simulink model "StateFlows_RevF"  (R2020a)
settings: Solver=FixedStepAuto  StartTime=0.0  StopTime=10.0  FixedStep=1e-3  RelTol=1e-3  EnableMultiTasking=on
undefined symbols (not defined in the file): A0, A1, D0, D1, D10, D11, D12, D13, D2, D3, D5, D6, D8, D9, PTA0, PTA1, PTA2, PTB2, PTB3, PTB9, PTC16, PTC17, PTC2, PTC4, PTD0, PTD1, PTD2, PTD3
libraries: frdmk64flib x17, etargetslib x13, dspstat3 x1
settings Model: ExtModeTrigDuration=5  Creator=dexho  LastModifiedBy=dexho
settings OptimizationCC: EnhancedBackFolding=on  PassReuseOutputArgsAs=Individual arguments  ZeroExternalMemoryAtStartup=off  ZeroInternalMemoryAtStartup=off  MaxStackSize=64  OptimizeBlockOrder=speed  DifferentSizesBufferReuse=on  OptimizationCustomize=off  EfficientTunableParamExpr=on
settings DebuggingCC: ParameterTunabilityLossMsg=error  UnconnectedInputMsg=none  UnconnectedOutputMsg=none  UnconnectedLineMsg=none
settings HardwareCC: ProdBitPerPointer=32  ProdBitPerSizeT=32  ProdBitPerPtrDiffT=32  ProdLargestAtomicInteger=Long  ProdLargestAtomicFloat=Double  ProdWordSize=32  ProdHWDeviceType=ARM Compatible->ARM Cortex
settings ModelReferenceCC: EnableRefExpFcnMdlSchedulingChecks=off
settings SFSimCC: MATLABDynamicMemAlloc=off
settings RTWCC: SystemTargetFile=ert.tlc  HardwareBoard=NXP FRDM-K64F  TemplateMakefile=ert_default_tmf  Toolchain=GNU Tools for ARM Embedded Processors
settings CodeAppCC: ForceParamTrailComments=on  IgnoreCustomStorageClasses=off  OperatorAnnotations=on  SimulinkDataObjDesc=on  SFDataObjDesc=on  InsertBlockDesc=on
settings ERTTargetCC: ExtModeTransport=4  ExtModeMexFile=sendToCommService

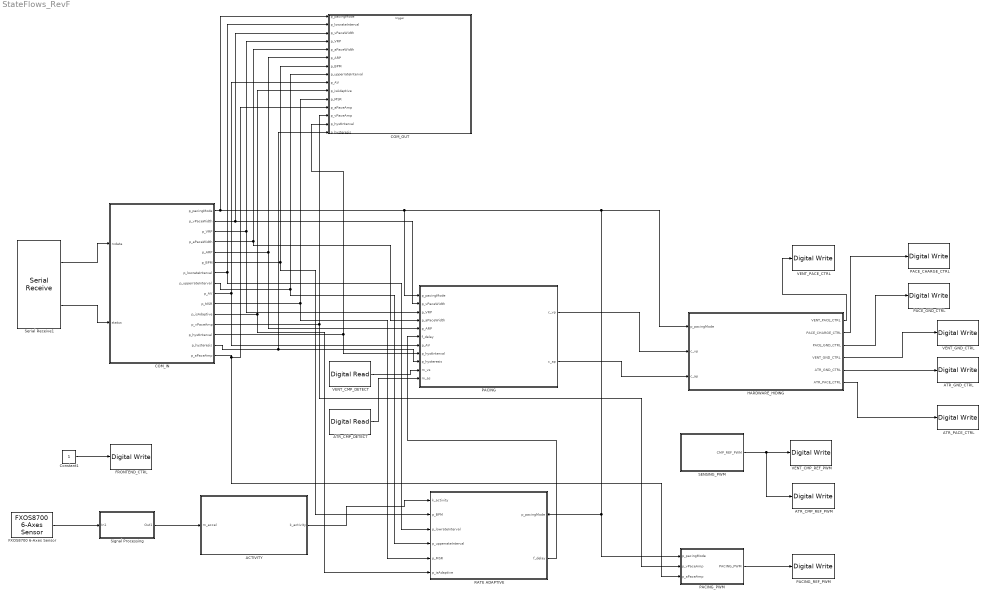
== system StateFlows_RevF ==
  ACTIVITY : Stateflow chart  TreatAsAtomicUnit=on
  ATR_CMP_DETECT : frdmk64flib/Digital Read  Whichpin=PTC16 (D0)  SampleTime=-1
  ATR_CMP_REF_PWM : frdmk64flib/Digital Write  Whichpin=PTC2 (D6)
  ATR_GND_CTRL : frdmk64flib/Digital Write  Whichpin=PTD2 (D11)
  ATR_PACE_CTRL : frdmk64flib/Digital Write  Whichpin=PTA0 (D8)
  COM_IN : Stateflow chart  TreatAsAtomicUnit=on
      settings: PortSchema="{\"entries\":[{\"content\":{\"sides\":[{\"content\":{\"connectorIds\":[\"In1\",\"In2\"]},\"type\":\"ConnectorPlacement.EquallySpacedRectSide\",\"uuid\":\"4343c62c-52df-4cc9-ac4a-2b1e5390f7dd\"},{\"content\":{\"connectorIds\":[\"Out1\",\"Out3\",\"Out4\",\"Out5\",\"Out6\",\"Out7\",\"Out2\",\"Out8\",\"Out9\",\"Out11\",\"Out10\",\"Out13\",\"Out14\",\"Out15\",\"Out12\"],\"side\":\"RIGHT\"},\"type\":\"ConnectorPlacement.EquallySpacedRectSide\",\"uuid\":\"27c89a21-e9bb-4d00-a5b8-19e687f961a4\"},{\"content\":{\"connectorIds\":[],\"side\":\"TOP\"},\"type\":\"ConnectorPlacement.EquallySpacedRectSide\",\"uuid\":\"0da42faa-8fe8-4994-9d32-ed3ce1a64f57\"}]},\"type\":\"ConnectorPlacement.EquallySpacedConnector\",\"uuid\":\"30cce4c4-f2f2-4d0d-92ef-56531670e1a1\"}],\"packageUris\":[\"http://schema.mathworks.com/mf0/Connector/19700101\"],\"version\":\"1.0\"}"
  COM_OUT : Subsystem
  Constant1 : Constant
  FRONTEND_CTRL : frdmk64flib/Digital Write  Whichpin=PTD1 (D13)
  FXOS8700 6-Axes Sensor : frdmk64flib/FXOS8700 6-Axes Sensor  Activesensor=Accelerometer only  ODR=100Hz  HybridODR=400Hz  Accelfullrange=-4g to +4g  SampleTime=-1
  HARDWARE_HIDING : Stateflow chart  TreatAsAtomicUnit=on
  PACE_CHARGE_CTRL : frdmk64flib/Digital Write  Whichpin=PTB9 (D2)
  PACE_GND_CTRL : frdmk64flib/Digital Write  Whichpin=PTD0 (D10)
  PACING : Stateflow chart  TreatAsAtomicUnit=on
      settings: PortSchema="{\"entries\":[{\"content\":{\"sides\":[{\"content\":{\"connectorIds\":[\"In3\",\"In4\",\"In5\",\"In6\",\"In7\",\"In8\",\"In9\",\"In10\",\"In11\",\"In1\",\"In2\"]},\"type\":\"ConnectorPlacement.EquallySpacedRectSide\",\"uuid\":\"abf03a48-0fa7-45c4-991f-e42ac80c6e9f\"},{\"content\":{\"connectorIds\":[\"Out1\",\"Out2\"],\"side\":\"RIGHT\"},\"type\":\"ConnectorPlacement.EquallySpacedRectSide\",\"uuid\":\"03e9df7b-3413-4ae5-9bc1-782036bbbe85\"},{\"content\":{\"connectorIds\":[],\"side\":\"TOP\"},\"type\":\"ConnectorPlacement.EquallySpacedRectSide\",\"uuid\":\"2119f2bc-1283-45d3-ae9d-33c8aada0ca6\"}]},\"type\":\"ConnectorPlacement.EquallySpacedConnector\",\"uuid\":\"89ff8e32-b874-4b74-b5d9-0aa878838f6d\"}],\"packageUris\":[\"http://schema.mathworks.com/mf0/Connector/19700101\"],\"version\":\"1.0\"}"
  PACING_PWM : Stateflow chart  TreatAsAtomicUnit=on
  PACING_REF_PWM : frdmk64flib/Digital Write  Whichpin=PTA2 (D5)
  RATE ADAPTIVE : Stateflow chart  TreatAsAtomicUnit=on
      settings: PortSchema="{\"entries\":[{\"content\":{\"sides\":[{\"content\":{\"connectorIds\":[\"In1\",\"In2\",\"In3\",\"In5\",\"In6\",\"In7\"]},\"type\":\"ConnectorPlacement.EquallySpacedRectSide\",\"uuid\":\"970c8990-33da-4b83-8419-4bdc08160303\"},{\"content\":{\"connectorIds\":[\"In4\",\"Out1\"],\"side\":\"RIGHT\"},\"type\":\"ConnectorPlacement.EquallySpacedRectSide\",\"uuid\":\"a18c4a49-244c-415b-8dfc-e199cb33ce07\"},{\"content\":{\"side\":\"TOP\"},\"type\":\"ConnectorPlacement.EquallySpacedRectSide\",\"uuid\":\"633c22bc-82ca-4f35-91f5-3ea1e9c4e467\"}]},\"type\":\"ConnectorPlacement.EquallySpacedConnector\",\"uuid\":\"9415645b-fdd6-4720-89a1-dcdad790b939\"}],\"packageUris\":[\"http://schema.mathworks.com/mf0/Connector/R2020b\"],\"version\":\"1.0\"}"
  SENSING_PWM : Stateflow chart  TreatAsAtomicUnit=on
  Serial Receive1 : frdmk64flib/Serial Receive  SCIModule=0  Baudrate=uint32(9600)  Parity=None  StopBits=1  HardwareFlowControl=None  ByteOrder=LittleEndian  DataType=uint8  DataLength=46  BlockingMode=off  OutputStatus=on  SampleTime=-1
  Signal Processing : Subsystem
  VENT_CMP_DETECT : frdmk64flib/Digital Read  Whichpin=PTC17 (D1)  SampleTime=-1
  VENT_CMP_REF_PWM : frdmk64flib/Digital Write  Whichpin=PTA1 (D3)
  VENT_GND_CTRL : frdmk64flib/Digital Write  Whichpin=PTD3 (D12)
  VENT_PACE_CTRL : frdmk64flib/Digital Write  Whichpin=PTC4 (D9)
  wires:
  VENT_CMP_DETECT/1 -> PACING/1(m_vs)
  ATR_CMP_DETECT/1 -> PACING/2(m_as)
  Constant1/1 -> FRONTEND_CTRL/1
  PACING_PWM/1(PACING_PWM) -> PACING_REF_PWM/1
  SENSING_PWM/1(CMP_REF_PWM) -> ATR_CMP_REF_PWM/1, VENT_CMP_REF_PWM/1
  COM_IN/1(p_pacingMode) -> COM_OUT/1(p_pacingMode), PACING/3(p_pacingMode), HARDWARE_HIDING/1(p_pacingMode), PACING_PWM/1(p_pacingMode), RATE ADAPTIVE/4(p_pacingMode)
  PACING/1(c_vp) -> HARDWARE_HIDING/2(c_vp)
  PACING/2(c_ap) -> HARDWARE_HIDING/3(c_ap)
  HARDWARE_HIDING/1(VENT_PACE_CTRL) -> VENT_PACE_CTRL/1
  HARDWARE_HIDING/2(PACE_CHARGE_CTRL) -> PACE_CHARGE_CTRL/1
  HARDWARE_HIDING/3(PACE_GND_CTRL) -> PACE_GND_CTRL/1
  HARDWARE_HIDING/4(VENT_GND_CTRL) -> VENT_GND_CTRL/1
  HARDWARE_HIDING/5(ATR_GND_CTRL) -> ATR_GND_CTRL/1
  HARDWARE_HIDING/6(ATR_PACE_CTRL) -> ATR_PACE_CTRL/1
  Signal Processing/1(Out1) -> ACTIVITY/1(m_accel)
  FXOS8700 6-Axes Sensor/1 -> Signal Processing/1(In1)
  ACTIVITY/1(k_activity) -> RATE ADAPTIVE/1(k_activity)
  RATE ADAPTIVE/1(f_delay) -> PACING/8(f_delay)
  Serial Receive1/1 -> COM_IN/1(rxdata)
  Serial Receive1/2 -> COM_IN/2(status)
  COM_IN/3(p_vPaceWidth) -> COM_OUT/3(p_vPaceWidth), PACING/4(p_vPaceWidth)
  COM_IN/4(p_VRP) -> PACING/5(p_VRP), COM_OUT/4(p_VRP)
  COM_IN/5(p_aPaceWidth) -> PACING/6(p_aPaceWidth), COM_OUT/5(p_aPaceWidth)
  COM_IN/6(p_ARP) -> PACING/7(p_ARP), COM_OUT/6(p_ARP)
  COM_IN/9(p_AV) -> PACING/9(p_AV), COM_OUT/9(p_AV)
  COM_IN/11(p_MSR) -> RATE ADAPTIVE/6(p_MSR), COM_OUT/11(p_MSR)
  COM_IN/10(p_isAdaptive) -> RATE ADAPTIVE/7(p_isAdaptive), COM_OUT/10(p_isAdaptive)
  COM_IN/8(p_upperrateInterval) -> RATE ADAPTIVE/5(p_upperrateInterval), COM_OUT/8(p_upperrateInterval)
  COM_IN/2(p_lowrateInterval) -> RATE ADAPTIVE/3(p_lowrateInterval), COM_OUT/2(p_lowrateInterval)
  COM_IN/7(p_BPM) -> RATE ADAPTIVE/2(p_BPM), COM_OUT/7(p_BPM)
  COM_IN/13(p_vPaceAmp) -> PACING_PWM/2(p_vPaceAmp), COM_OUT/13(p_vPaceAmp)
  COM_IN/12(p_aPaceAmp) -> PACING_PWM/3(p_aPaceAmp), COM_OUT/12(p_aPaceAmp)
  COM_IN/14(p_hystInterval) -> PACING/10(p_hystInterval), COM_OUT/14(p_hystInterval)
  COM_IN/15(p_hysteresis) -> COM_OUT/15(p_hysteresis), PACING/11(p_hysteresis)

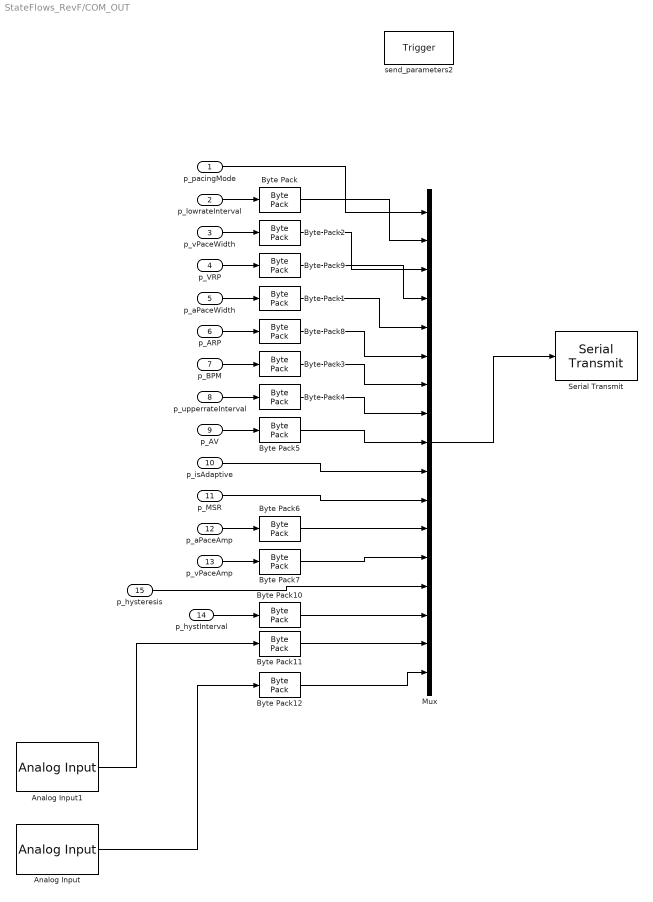
== system StateFlows_RevF/COM_OUT ==
  p_pacingMode : Inport  OutDataTypeStr=uint8
  p_lowrateInterval : Inport  Port=2  OutDataTypeStr=single
  p_vPaceWidth : Inport  Port=3  OutDataTypeStr=single
  p_VRP : Inport  Port=4  OutDataTypeStr=uint16
  p_aPaceWidth : Inport  Port=5  OutDataTypeStr=single
  p_ARP : Inport  Port=6  OutDataTypeStr=uint16
  p_BPM : Inport  Port=7  OutDataTypeStr=single
  p_upperrateInterval : Inport  Port=8  OutDataTypeStr=single
  p_AV : Inport  Port=9  OutDataTypeStr=single
  p_isAdaptive : Inport  Port=10  OutDataTypeStr=uint8
  p_MSR : Inport  Port=11  OutDataTypeStr=uint8
  p_aPaceAmp : Inport  Port=12  OutDataTypeStr=single
  p_vPaceAmp : Inport  Port=13  OutDataTypeStr=single
  p_hystInterval : Inport  Port=14  OutDataTypeStr=single
  p_hysteresis : Inport  Port=15  OutDataTypeStr=uint8
  send_parameters2 : TriggerPort  TriggerType=function-call  IsSimulinkFunction=on  FunctionName=send_parameters2  VariantControl=(inherit)  PortDimensions=1
  Analog Input : frdmk64flib/Analog Input  Whichpin=PTB2 (A0)  SampleTime=-1
  Analog Input1 : frdmk64flib/Analog Input  Whichpin=PTB3 (A1)  SampleTime=-1
  Byte Pack{,1..7,10} (9 alike) : etargetslib/Byte Pack  datatypes={'single'}  byteAlign=1
  Byte Pack11 : etargetslib/Byte Pack  datatypes={'double'}  byteAlign=1
  Byte Pack12 : etargetslib/Byte Pack  datatypes={'double'}  byteAlign=1
  Byte Pack8 : etargetslib/Byte Pack  datatypes={'uint16'}  byteAlign=1
  Byte Pack9 : etargetslib/Byte Pack  datatypes={'uint16'}  byteAlign=1
  Mux : Mux  Inputs=17
  Serial Transmit : frdmk64flib/Serial Transmit  SCIModule=0  Baudrate=uint32(9600)  Parity=None  StopBits=1  HardwareFlowControl=None  ByteOrder=LittleEndian  BlockingMode=on  OutputStatus=off
  wires:
  Mux/1 -> Serial Transmit/1
  p_pacingMode/1 -> Mux/1
  p_lowrateInterval/1 -> Byte Pack/1
  p_vPaceWidth/1 -> Byte Pack2/1
  p_VRP/1 -> Byte Pack9/1
  p_aPaceWidth/1 -> Byte Pack1/1
  p_ARP/1 -> Byte Pack8/1
  p_BPM/1 -> Byte Pack3/1
  p_upperrateInterval/1 -> Byte Pack4/1
  p_AV/1 -> Byte Pack5/1
  p_aPaceAmp/1 -> Byte Pack6/1
  p_vPaceAmp/1 -> Byte Pack7/1
  Byte Pack/1 -> Mux/2
  Byte Pack2/1 -> Mux/3
  Byte Pack9/1 -> Mux/4
  Byte Pack1/1 -> Mux/5
  Byte Pack8/1 -> Mux/6
  Byte Pack3/1 -> Mux/7
  Byte Pack4/1 -> Mux/8
  Byte Pack5/1 -> Mux/9
  p_isAdaptive/1 -> Mux/10
  p_MSR/1 -> Mux/11
  Byte Pack6/1 -> Mux/12
  Byte Pack7/1 -> Mux/13
  p_hystInterval/1 -> Byte Pack10/1
  Byte Pack10/1 -> Mux/15
  Byte Pack11/1 -> Mux/16
  Byte Pack12/1 -> Mux/17
  Analog Input/1 -> Byte Pack12/1
  Analog Input1/1 -> Byte Pack11/1
  p_hysteresis/1 -> Mux/14

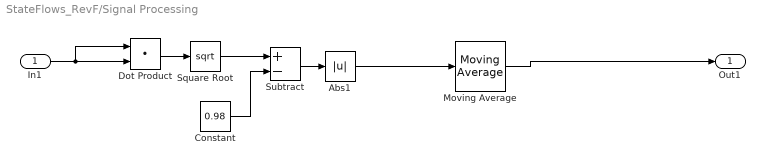
== system StateFlows_RevF/Signal Processing ==
  In1 : Inport
  Abs1 : Abs  OutDataTypeStr=double
  Constant : Constant  Value=0.98  OutDataTypeStr=double
  Dot Product : DotProduct  OutDataTypeStr=double  InputSameDT=on
  Moving Average : dspstat3/Moving Average  Method=Exponential weighting  ForgettingFactorPort=off  SpecifyWindowLength=on  WindowLength=4  ForgettingFactor=0.94  SimulateUsing=Code generation
  Square Root : Sqrt  OutputSignalType=real  OutDataTypeStr=double  SaturateOnIntegerOverflow=on
  Subtract : Sum  Inputs=+-
  Out1 : Outport  OutDataTypeStr=double
  wires:
  Constant/1 -> Subtract/2
  In1/1 -> Dot Product/2, Dot Product/1
  Subtract/1 -> Abs1/1
  Square Root/1 -> Subtract/1
  Dot Product/1 -> Square Root/1
  Abs1/1 -> Moving Average/1
  Moving Average/1 -> Out1/1

== stateflow chart StateFlows_RevF/SENSING_PWM ==
  state ON
    entry:
    CMP_REF_PWM = true;
  state OFF
    entry:
    CMP_REF_PWM = false;
  (default) -> ON
  ON -> OFF : [after((1000/freq)*0.8, msec)]
  OFF -> ON : [after((1000/freq)*0.2, msec)]
  data: CMP_REF_PWM output boolean; freq local double =200

== stateflow chart StateFlows_RevF/PACING_PWM ==
  state INIT
    entry:
    if(p_pacingMode == 0 || p_pacingMode == 2)
    f_dc = p_vPaceAmp / 5000;
    else
    f_dc = p_aPaceAmp / 5000;
    end
  state ON
    entry:
    PACING_PWM = true;
  state OFF
    entry:
    PACING_PWM = false;
  (default) -> INIT
  INIT -> ON
  ON -> OFF : [after((1000.0/freq)*f_dc, msec)]
  OFF -> ON : [after((1000.0/freq)*(1 - f_dc), msec)]
  data: PACING_PWM output boolean; freq local double =2000; p_pacingMode input uint8; p_vPaceAmp input single; p_aPaceAmp input single; f_dc local

== stateflow chart StateFlows_RevF/PACING ==
  state INIT
    entry:
    k_isHyst = 0;
  state CHARGE_DISCHARGE
    entry:
    c_vp = false;
    c_ap = false;
    if(p_pacingMode == 0 || p_pacingMode == 2)
    f_paceWidth = p_vPaceWidth;
    else
    f_paceWidth = p_aPaceWidth;
    end
    if(p_hysteresis == 0)
    k_isHyst = 0
    end
  state PACE
    entry:
  state DDD_vPace
    entry:
  state DDD_vSense
    entry:
  state DDD_aSense
    entry:
  state V_WAIT
    entry:
  state DDD_A
    entry:
  state DDD_V
    entry:
  state DDD_aPace
    entry:
  state A_WAIT
    entry:
  state VRP
    entry:
    if(p_hysteresis)
    k_isHyst = 1
    end
  state V_SENSE
    entry:
  state ARP
    entry:
    if(p_hysteresis)
    k_isHyst = 1
    end
  state A_SENSE
    entry:
  (default) -> INIT
  (junction 119) -> INIT
  (junction 114) -> INIT
  INIT -> CHARGE_DISCHARGE
  (junction 105) -> CHARGE_DISCHARGE
  PACE -> CHARGE_DISCHARGE : [after(f_paceWidth, msec)]
  CHARGE_DISCHARGE -> CHARGE_DISCHARGE [order 2] : [p_pacingMode == 4]
  DDD_vPace -> (junction 105) : [after(p_vPaceWidth, msec)]{c_vp = false}
  DDD_vSense -> (junction 105) [order 1] : [~m_vs]
  V_WAIT -> PACE : [after(f_delay - p_vPaceWidth, msec)]{c_vp = true}
  DDD_vSense -> (junction 119) [order 2] : [p_pacingMode ~= 5]
  DDD_aSense -> (junction 119) [order 2] : [p_pacingMode ~= 5]
  ARP -> PACE [order 2] : [after(f_delay + k_isHyst * p_hystInterval, msec)]{c_ap = true}
  A_SENSE -> PACE [order 2] : [after(f_delay - p_aPaceWidth + k_isHyst * p_hystInterval, msec)]{c_ap = true}
  VRP -> PACE [order 2] : [after(f_delay + k_isHyst * p_hystInterval, msec)]{c_vp = true}
  V_SENSE -> PACE [order 1] : [after(f_delay - p_vPaceWidth + k_isHyst * p_hystInterval, msec)]{c_vp = true}
  A_WAIT -> PACE : [after(f_delay - p_aPaceWidth, msec)]{c_ap = true}
  CHARGE_DISCHARGE -> (junction 42) [order 1]
  DDD_V -> DDD_vPace [order 2] : [after(p_AV, msec)]{c_vp = true}
  DDD_V -> DDD_vSense [order 1] : [m_vs]
  DDD_A -> DDD_aSense [order 1] : [m_as]
  DDD_aSense -> DDD_V [order 1] : [~m_as]
  (junction 42) -> A_SENSE [order 3] : [p_pacingMode == 3]
  (junction 42) -> DDD_A [order 5] : [p_pacingMode == 5]
  (junction 42) -> V_WAIT [order 4] : [(p_pacingMode == 0)]
  (junction 42) -> A_WAIT [order 1] : [(p_pacingMode == 1)]
  (junction 42) -> V_SENSE [order 2] : [p_pacingMode == 2]
  DDD_aPace -> DDD_V : [after(p_aPaceWidth, msec)]{c_ap = false}
  DDD_A -> DDD_aPace [order 2] : [after(f_delay - p_aPaceWidth - p_vPaceWidth - p_AV, msec)]{c_ap = true}
  VRP -> VRP [order 1] : [m_vs]
  VRP -> (junction 114) [order 3] : [p_pacingMode ~= 2]
  V_SENSE -> VRP [order 2] : [m_vs]
  ARP -> (junction 114) [order 3] : [p_pacingMode ~= 3]
  ARP -> ARP [order 1] : [m_as]
  A_SENSE -> ARP [order 1] : [m_as]{k_isHyst = 1}
  data: m_vs input boolean; m_as input boolean; c_vp output boolean =false; c_ap output boolean =false; p_pacingMode input uint8; p_vPaceWidth input single; p_VRP input uint16; p_aPaceWidth input single; p_ARP input uint16; f_paceWidth local single; f_delay input single =1000; p_AV input single; p_hystInterval input single; k_isHyst local single; p_hysteresis input uint8

== stateflow chart StateFlows_RevF/HARDWARE_HIDING ==
  state INIT
    entry:
    k_wasVent = 0;
    VENT_PACE_CTRL = 0;
    PACE_CHARGE_CTRL = 0;
    PACE_GND_CTRL = 0;
    VENT_GND_CTRL = 0;
    ATR_GND_CTRL = 0;
    ATR_PACE_CTRL = 0;
  state CHARGE_DISCHARGE
    entry:
    PACE_CHARGE_CTRL = 1;
    PACE_GND_CTRL = 1;
    if((p_pacingMode == 0) || (p_pacingMode == 2))
    VENT_PACE_CTRL = 0;
    VENT_GND_CTRL = 1;
    ATR_PACE_CTRL = 0;
    ATR_GND_CTRL = 0;
    elseif((p_pacingMode == 1) || (p_pacingMode == 3))
    VENT_PACE_CTRL = 0;
    VENT_GND_CTRL = 0;
    ATR_PACE_CTRL = 0;
    ATR_GND_CTRL = 1;
    else
    VENT_PACE_CTRL = 0;
    ATR_PACE_CTRL = 0;
    if(k_wasVent)
    VENT_GND_CTRL = 1;
    ATR_GND_CTRL = 0;
    else
    ATR_GND_CTRL = 1;
    VENT_GND_CTRL = 0;
    end
    end
  state VENT_PACE
    entry:
    PACE_CHARGE_CTRL = 0;
    VENT_PACE_CTRL = 1;
    VENT_GND_CTRL = 0;
    k_wasVent = 1;
  state ATR_PACE
    entry:
    PACE_CHARGE_CTRL = 0;
    ATR_PACE_CTRL = 1;
    ATR_GND_CTRL = 0;
    k_wasVent = 0;
  (default) -> INIT
  INIT -> CHARGE_DISCHARGE
  VENT_PACE -> CHARGE_DISCHARGE : [~c_vp]
  CHARGE_DISCHARGE -> VENT_PACE [order 1] : [c_vp]{ATR_GND_CTRL = 0}
  CHARGE_DISCHARGE -> ATR_PACE [order 2] : [c_ap]{VENT_GND_CTRL = 0}
  ATR_PACE -> CHARGE_DISCHARGE : [~c_ap]
  data: p_pacingMode input uint8; c_vp input boolean; c_ap input boolean; VENT_PACE_CTRL output uint8; PACE_CHARGE_CTRL output uint8; PACE_GND_CTRL output uint8; VENT_GND_CTRL output uint8; ATR_GND_CTRL output uint8; ATR_PACE_CTRL output uint8; k_wasVent local uint8

== stateflow chart StateFlows_RevF/ACTIVITY ==
  state STILL
    entry:
    k_activity = 0;
  state SLOW
    entry:
    k_activity = 1;
  state init
    entry:
  state ACC_INIT
    entry:
    k_activity = 0;
  state MODERATE
    entry:
    k_activity = 2;
  state FAST
    entry:
    k_activity = 3;
  (junction 20) -> init
  STILL -> (junction 20)
  (junction 6) -> STILL [order 1] : [m_accel <= 0.05]
  (default) -> ACC_INIT
  (junction 6) -> SLOW [order 2] : [m_accel > 0.05 && m_accel <= 0.2]
  ACC_INIT -> init
  init -> (junction 6)
  (junction 6) -> MODERATE [order 4] : [m_accel > 0.2 && m_accel <= 0.5]
  (junction 6) -> FAST [order 3] : [m_accel > 0.5]
  SLOW -> (junction 20)
  MODERATE -> (junction 20)
  FAST -> (junction 20)
  data: m_accel input double; k_activity output uint8

== stateflow chart StateFlows_RevF/RATE ADAPTIVE ==
  state OTHER_TRANSFER
    entry:
  state DEC_BPM
    entry:
    k_BPMR = k_BPMR - 0.005
  state INIT
    entry:
    k_BPMR = p_BPM;
    f_delay = 60000 / p_BPM;
  state INTERMED
    entry:
  state TRANSFER
    entry:
  state INC_BPM
    entry:
    if(k_activity == 1)
    k_BPMR = k_BPMR + 0.005;
    elseif(k_activity == 2)
    k_BPMR = k_BPMR + 0.01;
    else
    k_BPMR = k_BPMR + 0.02;
    end
  state NOT_ADAPTIVE
    entry:
    %error catching
    if(f_delay > 60000/p_lowrateInterval) %too slow
    k_BPMR = p_lowrateInterval;
    elseif(f_delay < 60000/p_upperrateInterval) %too fast
    k_BPMR = k_BPMR - 0.005;
    elseif(k_BPMR > p_BPM)
    k_BPMR = k_BPMR - 0.005;
    elseif(k_BPMR < p_BPM)
    k_BPMR = k_BPMR + 0.005;
    end
    f_delay = 60000/k_BPMR
  (default) -> INIT
  INTERMED -> OTHER_TRANSFER [order 1] : [k_activity == 0]
  OTHER_TRANSFER -> DEC_BPM [order 2]
  DEC_BPM -> (junction 72)
  OTHER_TRANSFER -> INC_BPM [order 1] : [(k_BPMR) <= p_lowrateInterval]
  INIT -> (junction 12)
  (junction 12) -> INTERMED [order 2]
  TRANSFER -> INC_BPM [order 2]
  (junction 17) -> (junction 12)
  INTERMED -> TRANSFER [order 2]
  (junction 12) -> NOT_ADAPTIVE [order 1] : [~p_isAdaptive]
  TRANSFER -> (junction 17) [order 1] : [k_BPMR >= p_MSR]
  INC_BPM -> (junction 72)
  (junction 72) -> (junction 17) : [after(1, msec)]{f_delay = 60000/k_BPMR}
  NOT_ADAPTIVE -> (junction 17)
  data: k_activity input uint8; f_delay output single; p_BPM input single; p_lowrateInterval input single; p_pacingMode input uint8; p_upperrateInterval input single; k_BPMR local single; p_MSR input uint8; p_isAdaptive input uint8

== stateflow chart StateFlows_RevF/COM_IN ==
  settings: executeAtInitialization=1
  state SET_PARAM
    entry:
    p_pacingMode = rxdata(3);
    p_lowrateInterval = typecast(rxdata(4:7), 'single');
    p_vPaceWidth = typecast(rxdata(8:11), 'single');
    p_VRP = typecast(rxdata(12:13), 'uint16');
    p_aPaceWidth = typecast(rxdata(14:17), 'single')
    p_ARP = typecast(rxdata(18:19), 'uint16');
    p_BPM = typecast(rxdata(20:23), 'single');
    p_upperrateInterval = typecast(rxdata(24:27), 'single');
    p_AV = typecast(rxdata(28:31), 'single')
    p_isAdaptive = rxdata(32)
    p_MSR = rxdata(33)
    p_aPaceAmp = typecast(rxdata(34:37), 'single')
    p_vPaceAmp = typecast(rxdata(38:41), 'single')
    p_hysteresis = rxdata(42)
    p_hystInterval = typecast(rxdata(43:46), 'single')
  state INITIAL
    % Initial values of parameters
    entry:
    p_pacingMode = 5;
    p_lowrateInterval = 60;
    p_vPaceWidth = 1.0;
    p_VRP = 320;
    p_aPaceWidth = 1.0;
    p_ARP = 250;
    p_BPM = 80;
    p_upperrateInterval = 120;
    p_AV = 150;
    p_isAdaptive = 1;
    p_MSR = 175;
    p_aPaceAmp = 3500;
    p_vPaceAmp = 3500;
    p_hysteresis = 0;
    p_hystInterval = 100;
  state STANDBY
    % Waiting for serial
  state ECHO_PARAM
    entry:
    send_parameters2();
  SET_PARAM -> STANDBY
  (default) -> INITIAL
  (junction 20) -> SET_PARAM [order 1] : [rxdata(2) == hex2dec('55')]
  (junction 17) -> STANDBY [order 2]
  INITIAL -> STANDBY
  STANDBY -> (junction 17) : [status == 0]
  (junction 17) -> (junction 20) [order 1] : [rxdata(1) == hex2dec('16')]
  (junction 20) -> ECHO_PARAM [order 2] : [rxdata(2) == hex2dec('22')]
  ECHO_PARAM -> STANDBY
  data: rxdata input uint8; status input uint8; p_pacingMode output uint8; p_lowrateInterval output single; p_vPaceWidth output single; p_VRP output uint16; p_aPaceWidth output single; p_ARP output uint16; p_BPM output single; p_upperrateInterval output single; p_AV output single; p_isAdaptive output uint8; p_MSR output uint8; p_aPaceAmp output single; p_vPaceAmp output single; p_hystInterval output single; p_hysteresis output uint8
